simulink model "ex2hybrid"  (R2020b)
settings: Solver=VariableStepAuto  StartTime=0.0  StopTime=5.0  RelTol=1e-3
values from neighbouring files (symbols this model uses):
  A1 = [-1 10;-100 -1]    [ex2.m]    (also in ex2runSimulink.m)
  A2 = [-1 100; -10 -1]    [ex2.m]    (also in ex2runSimulink.m)
  x10 = 1    [ex2runSimulink.m]
  x20 = 1    [ex2runSimulink.m]
settings Model: Creator=slacker  LastModifiedBy=slacker

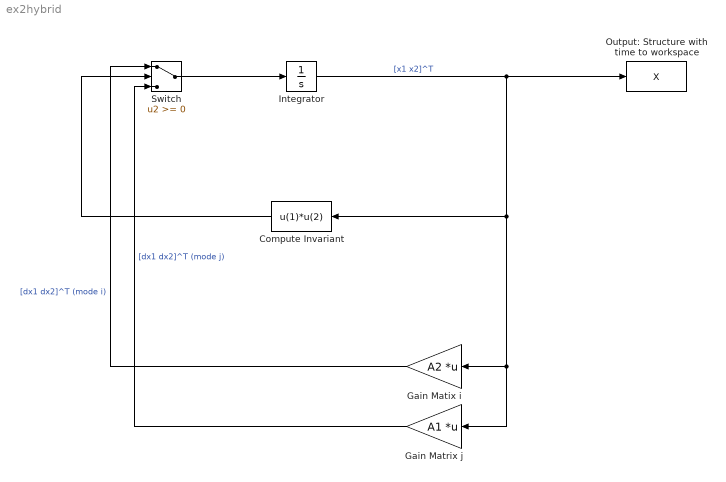
== system ex2hybrid ==
  Compute Invariant : Fcn  Expr=u(1)*u(2)
  Gain Matix i : Gain  Gain=A2  Multiplication=Matrix(K*u)
  Gain Matrix j : Gain  Gain=A1  Multiplication=Matrix(K*u)
  Integrator : Integrator  InitialCondition=[x10 x20]
  Output: Structure with time to workspace : ToWorkspace  VariableName=X  SaveFormat=Structure With Time  SampleTime=-1
  Switch : Switch
  wires:
  Gain Matrix j/1 -> Switch/3  "[dx1 dx2]^T (mode j)"
  Integrator/1 -> Output: Structure with time to workspace/1, Gain Matix i/1, Gain Matrix j/1, Compute Invariant/1  "[x1 x2]^T"
  Compute Invariant/1 -> Switch/2
  Switch/1 -> Integrator/1
  Gain Matix i/1 -> Switch/1  "[dx1 dx2]^T (mode i)"
